simulink model "lag"  (R2019a)
settings: Solver=VariableStepAuto  StartTime=0.0  StopTime=10.0  RelTol=1e-3
settings Model: Creator=amah2  LastModifiedBy=kovim

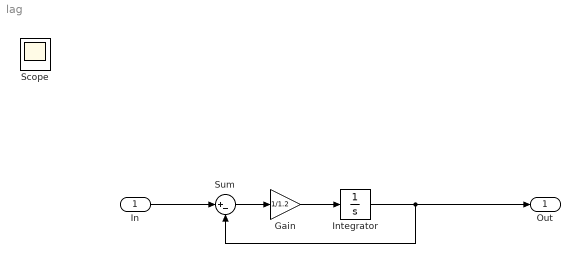
== system lag ==
  In : Inport
  Gain : Gain  Gain=1/1.2
  Integrator : Integrator
  Sum : Sum  Inputs=|+-
  Out : Outport
  Scope : Scope
  wires:
  In/1 -> Sum/1
  Gain/1 -> Integrator/1
  Sum/1 -> Gain/1
  Integrator/1 -> Sum/2, Out/1
